simulink model "Exemplo_Trabalho"  (R2022a)
settings: Solver=ode23tb  StartTime=0.0  StopTime=10  FixedStep=300e-6  MaxStep=1e-4  RelTol=1e-4
libraries: spsCurrentMeasurementLib x2, spsThreePhaseSeriesRLCLoadLib x1, spsGroundLib x1, spsThreePhaseSourceLib x1, spsSynchronousMachineSIFundamentalLib x1, spsVoltageMeasurementLib x1, spspowerguiLib x1
Description:
  | Copyright 2008-2019 The MathWorks, Inc.
settings Model: FPTRunName=Active  ExtModeTrigMode=oneshot  ExtModeArmWhenConnect=off  Creator=MathWorks  LastModifiedBy=marcone.faria
settings SolverCC: AlgebraicLoopSolver=TrustRegion
settings DataIOCC: InitialState=xFinal  SaveFormat=Array  SignalLoggingSaveFormat=ModelDataLogs  SaveOutput=off  ReturnWorkspaceOutputs=off  TimeSaveName=t  SignalLoggingName=sigsOut
settings OptimizationCC: BlockReduction=off  BooleanDataType=off  ExpressionDepthLimit=2147483647  InitFltsAndDblsToZero=on  EfficientMapNaN2IntZero=off  LifeSpan=inf
settings DebuggingCC: UnderspecifiedInitializationDetection=Classic  MergeDetectMultiDrivingBlocksExec=none  SignalResolutionControl=TryResolveAllWithWarning  MultiTaskDSMMsg=warning  MultiTaskCondExecSysMsg=none  SigSpecEnsureSampleTimeMsg=none  FcnCallInpInsideContextMsg=warning  UnconnectedLineMsg=warning  StateNameClashWarn=warning  SFUnexpectedBacktrackingDiag=warning  SFNoUnconditionalDefaultTransitionDiag=warning  SFExecutionAtInitializationDiag=none  SFMachineParentedDataDiag=warning  ArithmeticOperatorsInVariantConditions=warning
settings HardwareCC: ProdBitPerPointer=32  ProdBitPerSizeT=32  ProdBitPerPtrDiffT=32  ProdLargestAtomicFloat=None  ProdIntDivRoundTo=Undefined  ProdEndianess=Unspecified  ProdWordSize=32  ProdHWDeviceType=32-bit Generic  TargetUnknown=on
settings ModelReferenceCC: PropagateSignalLabelsOutOfModel=off
settings SFSimCC: SimUseLocalCustomCode=off  CustomCodeUndefinedFunction=UseInterfaceOnly
settings RTWCC: Description=Generic Real-Time Target  RTWUseLocalCustomCode=off
settings CodeAppCC: StateflowObjectComments=on
settings GRTTargetCC: TargetLangStandard=C89/C90 (ANSI)  CombineOutputUpdateFcns=off  GRTInterface=on
settings ConfigComp: CovMetricSettings=dw  CovSaveCumulativeToWorkspaceVar=on  CovSaveSingleToWorkspaceVar=on  CovExternalEMLEnable=off  CovSFcnEnable=off
settings SimscapeCC: SimscapeNormalizeSystem=off

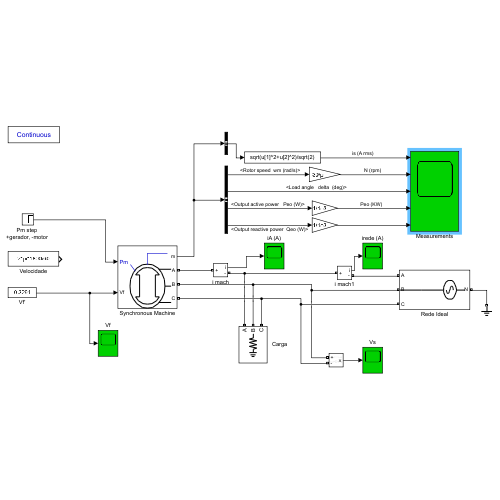
[thumbnail: Simulink's stored preview of the top-level diagram]
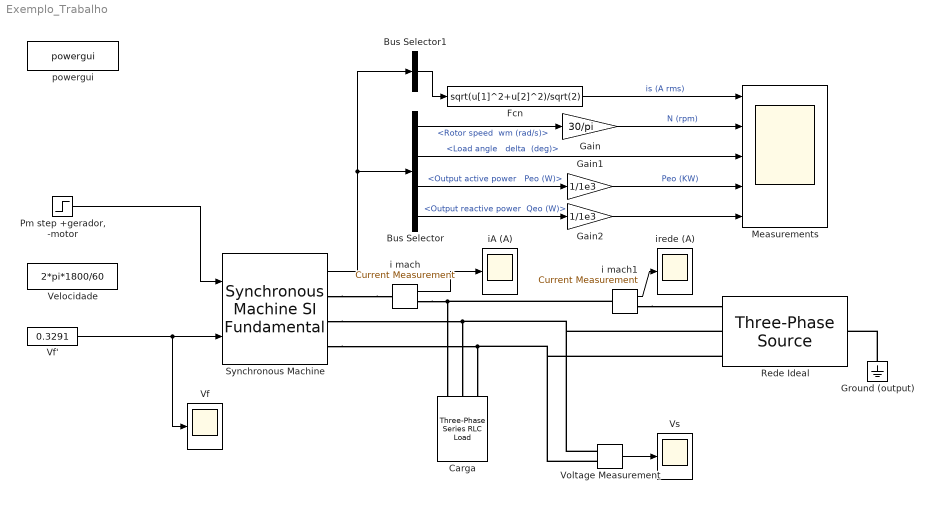
== system Exemplo_Trabalho ==
  " Carga" : spsThreePhaseSeriesRLCLoadLib/Three-Phase Series RLC Load  LConnTagsString=A|B|C  Configuration=Y (grounded)  NominalVoltage=460  Vabc=[1e3 1e3 1e3]  Vabcp=[1e3 1e3 1e3]  NominalFrequency=60  UnbalancedPower=off  ActivePower=2500e3*0.2  InductivePower=0  CapacitivePower=0  Pabc=[10e3 9e3 11e3]  QLabc=[100 90 110]  QCabc=[100 90 110]  Pabcp=[10e3 9e3 11e3]  QLabcp=[100 90 110]  QCabcp=[100 90 110]  Measurements=None  LoadType=constant PQ
  Bus Selector : BusSelector  OutputSignals="Mechanical.Rotor speed  wm (rad/s),Load angle   delta  (deg),Output active power   Peo (W),Output reactive power  Qeo (W)"
  Bus Selector1 : BusSelector  OutputSignals="dq0 components.Stator current  iq (A),dq0 components.Stator current  id (A)"  OutputAsBus=on
  Fcn : Fcn  Expr=sqrt(u[1]^2+u[2]^2)/sqrt(2)
  Gain : Gain  Gain=30/pi  SaturateOnIntegerOverflow=on  OutDataTypeStr=Inherit: Same as input  ParamDataTypeStr=Inherit: Same as input
  Gain1 : Gain  Gain=1/1e3  SaturateOnIntegerOverflow=on  OutDataTypeStr=Inherit: Same as input  ParamDataTypeStr=Inherit: Same as input
  Gain2 : Gain  Gain=1/1e3  SaturateOnIntegerOverflow=on  OutDataTypeStr=Inherit: Same as input  ParamDataTypeStr=Inherit: Same as input
  Ground (output) : spsGroundLib/Ground  LConnTagsString=a
  Measurements : Scope  NumInputPorts=5
  "Pm step +gerador, -motor " : Step  Time=2  After=2500e3*0.2  SampleTime=0
  "Rede Ideal " : spsThreePhaseSourceLib/Three-Phase Source  InternalConnection=Yn  VoltagePhases=off  Voltage=460  PhaseAngle=0  Voltage_phases=[25e3 25e3 25e3]/sqrt(3)  PhaseAngles_phases=[0 -120 +120]  Frequency=60  NonIdealSource=off  SpecifyImpedance=off  Resistance=762^2/10e6/10  Inductance=762^2/10e6/(2*pi*60)  ShortCircuitLevel=100e6  BaseVoltage=25e3  XRratio=7  BusType=swing  Pref=0  Qref=0  Prefabc=[10e3, 10e3, 10e3]  Qrefabc=[0, 0, 0]  Qmin=-Inf  Qmax=Inf
  Synchronous Machine : spsSynchronousMachineSIFundamentalLib/Synchronous Machine SI Fundamental  PresetModel=04: 50Hz 400V 42.5kVA 1500RPM  MechanicalLoad=Mechanical power Pm  ShowDetailedParameters=on  RotorType=Salient-pole  Units=SI fundamental parameters  MeasurementBus=off  NominalParameters=[4.25e+04 400 50]  Stator=[0.181 0.0009587 0.02529 0.01114]  Field=[0.1002 0.001895]  Dampers2=[ 1 2 3 4 5 6 ]  Dampers1=[0.2838 0.001316 0.2752 0.0007686]  Mechanical=[0.3987 0.033 2]  PolePairs=2  InitialConditions=[0 0 0 0 0 0 0 0 0.3291]  SetSaturation=off  Saturation=[46.376,51.647,61.167,66.773,72.147,78.393,86.24,95.347,105.58;644,708.2,816.2,870.87,917.13,962.47,1012,1059.3,1104.5]  DisplayVfd=off  LoadFlowParameters=[1 -50000 0 0 0]  TsPowergui=0  TsBlock=-1  IterativeModel=Trapezoidal non iterative  IterativeDiscreteModel=Trapezoidal non iterative  BusType=PV  Pref=-50000  Qref=0  Qmin=-Inf  Qmax=Inf  PLF=0  QLF=0
      settings: AttributesFormatString=\n  SourceProductBaseCode=PS
  Velocidade : Constant  Value=2*pi*1800/60
  Vf : Scope
  Vf' : Constant  Value=0.3291
  Voltage Measurement : spsVoltageMeasurementLib/Voltage Measurement  PhasorSimulation=off  OutputType=Complex  PSBequivalent=0
  Vs : Scope
  i mach : spsCurrentMeasurementLib/Current Measurement  Tag=PoWeRsYsTeMmEaSuReMeNt  PhasorSimulation=off  OutputType=Magnitude  PSBequivalent=0
      settings: AttributesFormatString=\n
  i mach1 : spsCurrentMeasurementLib/Current Measurement  Tag=PoWeRsYsTeMmEaSuReMeNt  PhasorSimulation=off  OutputType=Magnitude  PSBequivalent=0
      settings: AttributesFormatString=\n
  iA (A) : Scope
  irede (A) : Scope
  powergui : spspowerguiLib/powergui  Priority=2  SimulationMode=Continuous  SampleTime=0  frequency=60  Iterations=50  frequencyindice=60  Pbase=1e6  ErrMax=0.0001  UnitsV=V  UnitsW=kW  buscounter=0  FunctionMessages=off  echomessages=off  EnableUseOfTLC=off  CurrentSourceSwitches=off  DisableSnubberDevices=off  DisableRonSwitches=off  DisableVfSwitches=off  DisplayEquations=off  AutomaticDiscreteSolvers=off  SolverType=Tustin  Interpol=off  ExternalGateDelay=off  methode=off  Ts=0  x0status=blocks  SPID=on  SwTol=0  HookPort=off  NonlinearTolerance=0  nMaxIteration=15  ContinueOnMaxIteration=off  RestoreLinks=warning  ResistiveCurrentMeasurement=off  Frange=logspace(0,3,50)  Ylog=off  Xlog=off  ShowGrid=off  save=off  variable=ZData  structure=0  ZoomFFT=on  StartTime=0.0  cycles=2  DisplayStyle=off  fundamental=60  FreqAxis=off  MaxFrequency=1000  frequencyindicesteady=1  RmsSteady=1  display=off
  wires:
  Fcn/1 -> Measurements/1  "is (A rms)"
  Bus Selector1/1 -> Fcn/1
  Gain/1 -> Measurements/2  "N (rpm)"
  Gain1/1 -> Measurements/4  "Peo (KW)"
  Synchronous Machine/1 -> Bus Selector1/1, Bus Selector/1
  Vf'/1 -> Vf/1, Synchronous Machine/2
  i mach/1 -> iA (A)/1
  Bus Selector/3 -> Gain1/1  "<Output active power   Peo (W)>"
  Bus Selector/2 -> Measurements/3  "<Load angle   delta  (deg)>"
  Bus Selector/1 -> Gain/1  "<Rotor speed  wm (rad/s)>"
  Voltage Measurement/1 -> Vs/1
  Bus Selector/4 -> Gain2/1  "<Output reactive power  Qeo (W)>"
  Gain2/1 -> Measurements/5
  "Pm step +gerador, -motor "/1 -> Synchronous Machine/1
  i mach1/1 -> irede (A)/1
  connections:
  Synchronous Machine/RConn1 -- i mach/LConn1
  Ground (output)/LConn1 -- "Rede Ideal "/LConn1
  Synchronous Machine/RConn3 -- Voltage Measurement/LConn2 -- "Rede Ideal "/RConn3 -- " Carga"/LConn3
  Synchronous Machine/RConn2 -- Voltage Measurement/LConn1 -- "Rede Ideal "/RConn2 -- " Carga"/LConn2
  i mach/RConn1 -- i mach1/LConn1 -- " Carga"/LConn1
  i mach1/RConn1 -- "Rede Ideal "/RConn1
